simulink model "test"  (R2018b)
settings: Solver=VariableStepAuto  StartTime=0.0  StopTime=inf  RelTol=1e-3
undefined symbols (not defined in the file or in its folder): currentCFG_test_UR, UR
libraries: Tools x1, gtecHighspeedLib x1, gUSBamplib x1
settings Model: Creator=User  LastModifiedBy=User

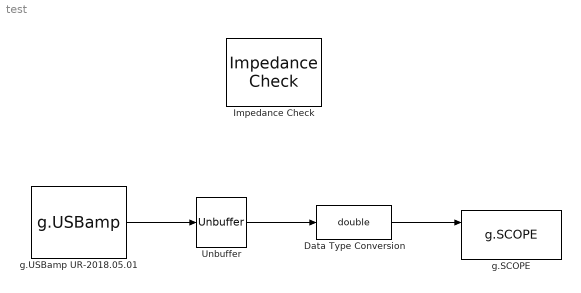
== system test ==
  Data Type Conversion : DataTypeConversion  OutDataTypeStr=double
  Impedance Check : Tools/Impedance Check
  Unbuffer : Unbuffer
  g.SCOPE : gtecHighspeedLib/g.SCOPE
      settings: SourceProductName=g.tec Highspeed Library
  g.USBamp UR-2018.05.01 : gUSBamplib/g.USBamp  cfg=currentCFG_test_UR-2018.05.01.cfg  snr=UR-2018.05.01
      settings: SourceProductName=g.USBamp
  wires:
  g.USBamp UR-2018.05.01/1 -> Unbuffer/1
  Unbuffer/1 -> Data Type Conversion/1
  Data Type Conversion/1 -> g.SCOPE/1
